simulink model "statefdbk"  (R2021a)
settings: Solver=VariableStepAuto  StartTime=0.0  StopTime=10.0  RelTol=1e-3
values from neighbouring files (symbols this model uses):
  K = lqr(A, B, Qr, Rr)    [lab1.m]    (also in lab1_observer.m; lab1_sim.m; matlab.mat = [-3.16227766017 -2.53239594036 22.2564178614 3.25706278131 0; varia_ganhos.m)
settings Model: Creator=afons  LastModifiedBy=afons

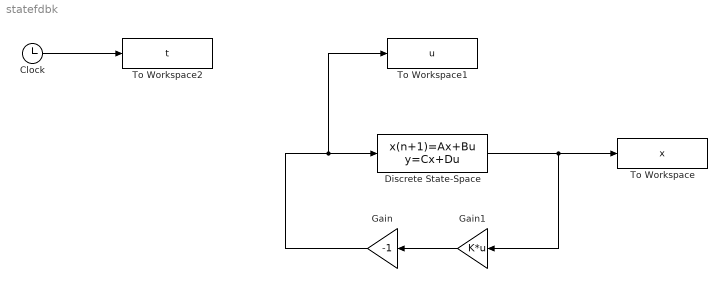
== system statefdbk ==
  Clock : Clock
  Discrete State-Space : DiscreteStateSpace  InitialCondition=1  SampleTime=-1
  Gain : Gain  Gain=-1
  Gain1 : Gain  Gain=K*u
  To Workspace : ToWorkspace  VariableName=x  SampleTime=-1
  To Workspace1 : ToWorkspace  VariableName=u  SampleTime=-1
  To Workspace2 : ToWorkspace  VariableName=t  SaveFormat=Timeseries  SampleTime=-1
  wires:
  Gain1/1 -> Gain/1
  Clock/1 -> To Workspace2/1
  Discrete State-Space/1 -> To Workspace/1, Gain1/1
  Gain/1 -> To Workspace1/1, Discrete State-Space/1
